simulink model "zad1"  (Simulink 7.3)
settings: Solver=ode45  StartTime=0.0  StopTime=10  MaxStep=0.01  RelTol=1e-3
settings Model: Creator=mklepacki  LastModifiedBy=mklepacki

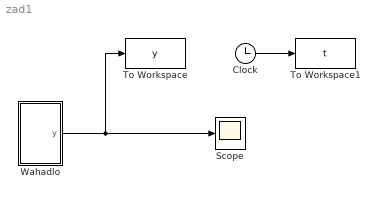
== system zad1 ==
  Clock : Clock
      settings: Decimation=10
  Scope : Scope
      settings: YMin=-0.6  YMax=1
  To Workspace : ToWorkspace  VariableName=y  SampleTime=-1  SaveFormat=Array
  To Workspace1 : ToWorkspace  VariableName=t  SampleTime=-1  SaveFormat=Array
  Wahadlo : Subsystem  mask{m=2, l=3, g=9.81, fi0=53, k=1}
      mask prompts: m "masa"; l "dlugosc"; g "przyspieszenie"; fi0 "kat"; k "wsp tlum"
  wires:
  Wahadlo/1(y) -> Scope/1, To Workspace/1
  Clock/1 -> To Workspace1/1

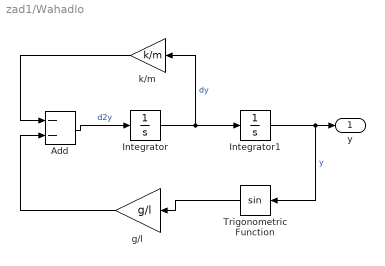
== system zad1/Wahadlo ==
  Add : Sum  Inputs=--  OutDataType=fixdt(1, 16)  OutScaling=2^-10
  Integrator : Integrator
  Integrator1 : Integrator  InitialCondition=fi0*pi/180
  Trigonometric Function : Trigonometry
  g/l : Gain  Gain=g/l  ParameterDataType=fixdt(1, 16)  ParameterScaling=2^0  OutDataType=fixdt(1, 16)  OutScaling=2^0
  k/m : Gain  Gain=k/m  ParameterDataType=fixdt(1, 16)  ParameterScaling=2^0  OutDataType=fixdt(1, 16)  OutScaling=2^0
  y : Outport
  wires:
  Add/1 -> Integrator/1  "d2y"
  Integrator/1 -> Integrator1/1, k/m/1  "dy"
  Integrator1/1 -> Trigonometric Function/1, y/1  "y"
  Trigonometric Function/1 -> g/l/1
  k/m/1 -> Add/1
  g/l/1 -> Add/2
